simulink model "case7"  (R2024b)
settings: Solver=FixedStepAuto  StartTime=0  StopTime=1  FixedStep=1e-7  RelTol=1e-3
values from neighbouring files (symbols this model uses):
  SG_D_1_D = 0.01056    [IEEE9_case_parameters.m]    (also in case1_parameters.m; case2_parameters.m; case3_parameters.m; case4_parameters.m)
  SG_D_1_EnableSaturation = 0    [IEEE9_case_parameters.m]    (also in case1_parameters.m; case2_parameters.m; case3_parameters.m; case4_parameters.m)
  SG_D_1_f0 = 60    [IEEE9_case_parameters.m]    (also in case1_parameters.m; case2_parameters.m; case3_parameters.m; case4_parameters.m)
  SG_D_1_H = 7.5    [IEEE9_case_parameters.m]    (also in case1_parameters.m; case2_parameters.m; case3_parameters.m; case4_parameters.m)
  SG_D_1_K_A = 20    [IEEE9_case_parameters.m]    (also in case1_parameters.m; case2_parameters.m; case3_parameters.m; case4_parameters.m)
  SG_D_1_K_E = 1.000000e+1    (= 10)    [IEEE9_case_parameters.m]    (also in case1_parameters.m; case2_parameters.m; case3_parameters.m; case4_parameters.m)
  SG_D_1_K_F = 2.363    [IEEE9_case_parameters.m]    (also in case1_parameters.m; case2_parameters.m; case3_parameters.m; case4_parameters.m)
  SG_D_1_K_s = 0.5    [IEEE9_case_parameters.m]    (also in case1_parameters.m = 5; case2_parameters.m = 5; case3_parameters.m = 5; case4_parameters.m = 5)
  SG_D_1_R_a = 0.001088    [IEEE9_case_parameters.m]    (also in case1_parameters.m; case2_parameters.m; case3_parameters.m; case4_parameters.m)
  SG_D_1_S_A = 1    [IEEE9_case_parameters.m]    (also in case1_parameters.m; case2_parameters.m; case3_parameters.m; case4_parameters.m)
  SG_D_1_S_B = 0.103    [IEEE9_case_parameters.m]    (also in case1_parameters.m; case2_parameters.m; case3_parameters.m; case4_parameters.m)
  SG_D_1_S_N = 10.659857    [IEEE9_case_parameters.m]    (also in case1_parameters.m; case2_parameters.m; case3_parameters.m; case4_parameters.m)
  SG_D_1_SpeedPara = 200    [IEEE9_case_parameters.m]    (also in case1_parameters.m; case2_parameters.m; case3_parameters.m; case4_parameters.m)
  SG_D_1_T_0 = 0.720173    [IEEE9_case_parameters.m]    (also in case1_parameters.m = 0.755522; case2_parameters.m = 0.808931; case3_parameters.m = 0.869402; case4_parameters.m = 0.729316)
  SG_D_1_T_1 = 0.3    [IEEE9_case_parameters.m]    (also in case1_parameters.m; case2_parameters.m; case3_parameters.m; case4_parameters.m)
  SG_D_1_T_2 = 0.05    [IEEE9_case_parameters.m]    (also in case1_parameters.m; case2_parameters.m; case3_parameters.m; case4_parameters.m)
  SG_D_1_T_3 = 0.02    [IEEE9_case_parameters.m]    (also in case1_parameters.m; case2_parameters.m; case3_parameters.m; case4_parameters.m)
  SG_D_1_T_4 = 0.005    [IEEE9_case_parameters.m]    (also in case1_parameters.m; case2_parameters.m; case3_parameters.m; case4_parameters.m)
  SG_D_1_T_A = 0.02    [IEEE9_case_parameters.m]    (also in case1_parameters.m; case2_parameters.m; case3_parameters.m; case4_parameters.m)
  SG_D_1_T_dd = 8.000000e+0    (= 8)    [IEEE9_case_parameters.m]    (also in case1_parameters.m; case2_parameters.m; case3_parameters.m; case4_parameters.m)
  SG_D_1_T_ddd = 0.04    [IEEE9_case_parameters.m]    (also in case1_parameters.m; case2_parameters.m; case3_parameters.m; case4_parameters.m)
  SG_D_1_T_E = 0.314    [IEEE9_case_parameters.m]    (also in case1_parameters.m; case2_parameters.m; case3_parameters.m; case4_parameters.m)
  SG_D_1_T_F = 0.35    [IEEE9_case_parameters.m]    (also in case1_parameters.m; case2_parameters.m; case3_parameters.m; case4_parameters.m)
  SG_D_1_T_qd = 0.8    [IEEE9_case_parameters.m]    (also in case1_parameters.m; case2_parameters.m; case3_parameters.m; case4_parameters.m)
  SG_D_1_T_qdd = 0.02    [IEEE9_case_parameters.m]    (also in case1_parameters.m; case2_parameters.m; case3_parameters.m; case4_parameters.m)
  SG_D_1_T_speed = 0.1    [IEEE9_case_parameters.m]    (also in case1_parameters.m = 200; case2_parameters.m = 200; case3_parameters.m = 200; case4_parameters.m = 200)
  SG_D_1_T_w = 0.5    [IEEE9_case_parameters.m]    (also in case1_parameters.m; case2_parameters.m; case3_parameters.m; case4_parameters.m)
  SG_D_1_V_ref = 1.990276    [IEEE9_case_parameters.m]    (also in case1_parameters.m = 2.042296; case2_parameters.m = 2.051388; case3_parameters.m = 2.089584; case4_parameters.m = 2.01845)
  SG_D_1_w_ref = 376.991118    [IEEE9_case_parameters.m]    (also in case1_parameters.m; case2_parameters.m; case3_parameters.m; case4_parameters.m)
  SG_D_1_wb = 6.000000e+1    (= 60)    [IEEE9_case_parameters.m]    (also in case1_parameters.m; case2_parameters.m; case3_parameters.m; case4_parameters.m)
  SG_D_1_x_d = 1.9    [IEEE9_case_parameters.m]    (also in case1_parameters.m; case2_parameters.m; case3_parameters.m; case4_parameters.m)
  SG_D_1_x_dd = 0.302    [IEEE9_case_parameters.m]    (also in case1_parameters.m; case2_parameters.m; case3_parameters.m; case4_parameters.m)
  SG_D_1_x_ddd = 0.204    [IEEE9_case_parameters.m]    (also in case1_parameters.m; case2_parameters.m; case3_parameters.m; case4_parameters.m)
  SG_D_1_x_l = 0.05    [IEEE9_case_parameters.m]    (also in case1_parameters.m; case2_parameters.m; case3_parameters.m; case4_parameters.m)
  SG_D_1_x_q = 1.3    [IEEE9_case_parameters.m]    (also in case1_parameters.m; case2_parameters.m; case3_parameters.m; case4_parameters.m)
  SG_D_1_x_qd = 0.5    [IEEE9_case_parameters.m]    (also in case1_parameters.m; case2_parameters.m; case3_parameters.m; case4_parameters.m)
  SG_D_1_x_qdd = 0.3    [IEEE9_case_parameters.m]    (also in case1_parameters.m; case2_parameters.m; case3_parameters.m; case4_parameters.m)
  SG_D_2_D = 0.02    [IEEE9_case_parameters.m]    (also in case1_parameters.m; case2_parameters.m; case3_parameters.m; case4_parameters.m)
  SG_D_2_EnableSaturation = 0    [IEEE9_case_parameters.m]    (also in case1_parameters.m; case2_parameters.m; case3_parameters.m; case4_parameters.m)
  SG_D_2_f0 = 60    [IEEE9_case_parameters.m]    (also in case1_parameters.m; case2_parameters.m; case3_parameters.m; case4_parameters.m)
  SG_D_2_H = 8.000000e+0    (= 8)    [IEEE9_case_parameters.m]    (also in case1_parameters.m; case2_parameters.m; case3_parameters.m; case4_parameters.m)
  SG_D_2_K_A = 20    [IEEE9_case_parameters.m]    (also in case1_parameters.m; case2_parameters.m; case3_parameters.m; case4_parameters.m)
  SG_D_2_K_E = 1.000000e+1    (= 10)    [IEEE9_case_parameters.m]    (also in case1_parameters.m; case2_parameters.m; case3_parameters.m; case4_parameters.m)
  SG_D_2_K_F = 2.363    [IEEE9_case_parameters.m]    (also in case1_parameters.m; case2_parameters.m; case3_parameters.m; case4_parameters.m)
  SG_D_2_K_s = 0.5    [IEEE9_case_parameters.m]    (also in case1_parameters.m = 4; case2_parameters.m = 4; case3_parameters.m = 4; case4_parameters.m = 4)
  SG_D_2_R_a = 0.001088    [IEEE9_case_parameters.m]    (also in case1_parameters.m; case2_parameters.m; case3_parameters.m; case4_parameters.m)
  SG_D_2_S_A = 1    [IEEE9_case_parameters.m]    (also in case1_parameters.m; case2_parameters.m; case3_parameters.m; case4_parameters.m)
  SG_D_2_S_B = 0.103    [IEEE9_case_parameters.m]    (also in case1_parameters.m; case2_parameters.m; case3_parameters.m; case4_parameters.m)
  SG_D_2_S_N = 10.659857    [IEEE9_case_parameters.m]    (also in case1_parameters.m; case2_parameters.m; case3_parameters.m; case4_parameters.m)
  SG_D_2_SpeedPara = 200    [IEEE9_case_parameters.m]    (also in case1_parameters.m; case2_parameters.m; case3_parameters.m; case4_parameters.m)
  SG_D_2_T_0 = 1.632913    [IEEE9_case_parameters.m]    (also in case1_parameters.m = 1.632925; case2_parameters.m = 1.632915; case3_parameters.m = 1.632914; case4_parameters.m = 1.632927)
  SG_D_2_T_1 = 0.2    [IEEE9_case_parameters.m]    (also in case1_parameters.m; case2_parameters.m; case3_parameters.m; case4_parameters.m)
  SG_D_2_T_2 = 0.05    [IEEE9_case_parameters.m]    (also in case1_parameters.m; case2_parameters.m; case3_parameters.m; case4_parameters.m)
  SG_D_2_T_3 = 0.02    [IEEE9_case_parameters.m]    (also in case1_parameters.m; case2_parameters.m; case3_parameters.m; case4_parameters.m)
  SG_D_2_T_4 = 0.005    [IEEE9_case_parameters.m]    (also in case1_parameters.m; case2_parameters.m; case3_parameters.m; case4_parameters.m)
  SG_D_2_T_A = 0.02    [IEEE9_case_parameters.m]    (also in case1_parameters.m; case2_parameters.m; case3_parameters.m; case4_parameters.m)
  SG_D_2_T_dd = 7.9    [IEEE9_case_parameters.m]    (also in case1_parameters.m; case2_parameters.m; case3_parameters.m; case4_parameters.m)
  SG_D_2_T_ddd = 0.04    [IEEE9_case_parameters.m]    (also in case1_parameters.m; case2_parameters.m; case3_parameters.m; case4_parameters.m)
  SG_D_2_T_E = 0.314    [IEEE9_case_parameters.m]    (also in case1_parameters.m; case2_parameters.m; case3_parameters.m; case4_parameters.m)
  SG_D_2_T_F = 0.35    [IEEE9_case_parameters.m]    (also in case1_parameters.m; case2_parameters.m; case3_parameters.m; case4_parameters.m)
  SG_D_2_T_qd = 0.8    [IEEE9_case_parameters.m]    (also in case1_parameters.m; case2_parameters.m; case3_parameters.m; case4_parameters.m)
  SG_D_2_T_qdd = 0.015    [IEEE9_case_parameters.m]    (also in case1_parameters.m; case2_parameters.m; case3_parameters.m; case4_parameters.m)
  SG_D_2_T_speed = 0.1    [IEEE9_case_parameters.m]    (also in case1_parameters.m = 150; case2_parameters.m = 150; case3_parameters.m = 150; case4_parameters.m = 150)
  SG_D_2_T_w = 0.35    [IEEE9_case_parameters.m]    (also in case1_parameters.m; case2_parameters.m; case3_parameters.m; case4_parameters.m)
  SG_D_2_V_ref = 2.58547    [IEEE9_case_parameters.m]    (also in case1_parameters.m = 2.597896; case2_parameters.m = 2.587136; case3_parameters.m = 2.586042; case4_parameters.m = 2.599679)
  SG_D_2_w_ref = 376.991118    [IEEE9_case_parameters.m]    (also in case1_parameters.m; case2_parameters.m; case3_parameters.m; case4_parameters.m)
  SG_D_2_wb = 6.000000e+1    (= 60)    [IEEE9_case_parameters.m]    (also in case1_parameters.m; case2_parameters.m; case3_parameters.m; case4_parameters.m)
  SG_D_2_x_d = 1.8    [IEEE9_case_parameters.m]    (also in case1_parameters.m; case2_parameters.m; case3_parameters.m; case4_parameters.m)
  SG_D_2_x_dd = 0.302    [IEEE9_case_parameters.m]    (also in case1_parameters.m; case2_parameters.m; case3_parameters.m; case4_parameters.m)
  SG_D_2_x_ddd = 0.204    [IEEE9_case_parameters.m]    (also in case1_parameters.m; case2_parameters.m; case3_parameters.m; case4_parameters.m)
  SG_D_2_x_l = 0.05    [IEEE9_case_parameters.m]    (also in case1_parameters.m; case2_parameters.m; case3_parameters.m; case4_parameters.m)
  SG_D_2_x_q = 1.25    [IEEE9_case_parameters.m]    (also in case1_parameters.m; case2_parameters.m; case3_parameters.m; case4_parameters.m)
  SG_D_2_x_qd = 0.5    [IEEE9_case_parameters.m]    (also in case1_parameters.m; case2_parameters.m; case3_parameters.m; case4_parameters.m)
  SG_D_2_x_qdd = 0.3    [IEEE9_case_parameters.m]    (also in case1_parameters.m; case2_parameters.m; case3_parameters.m; case4_parameters.m)
  SG_D_3_D = 0.02    [IEEE9_case_parameters.m]    (also in case1_parameters.m; case2_parameters.m; case3_parameters.m; case4_parameters.m)
  SG_D_3_EnableSaturation = 0    [IEEE9_case_parameters.m]    (also in case1_parameters.m; case2_parameters.m; case3_parameters.m; case4_parameters.m)
  SG_D_3_f0 = 60    [IEEE9_case_parameters.m]    (also in case1_parameters.m; case2_parameters.m; case3_parameters.m; case4_parameters.m)
  SG_D_3_H = 7.7    [IEEE9_case_parameters.m]    (also in case1_parameters.m; case2_parameters.m; case3_parameters.m; case4_parameters.m)
  SG_D_3_K_A = 20    [IEEE9_case_parameters.m]    (also in case1_parameters.m; case2_parameters.m; case3_parameters.m; case4_parameters.m)
  SG_D_3_K_E = 1.000000e+1    (= 10)    [IEEE9_case_parameters.m]    (also in case1_parameters.m; case2_parameters.m; case3_parameters.m; case4_parameters.m)
  SG_D_3_K_F = 2.363    [IEEE9_case_parameters.m]    (also in case1_parameters.m; case2_parameters.m; case3_parameters.m; case4_parameters.m)
  SG_D_3_K_s = 0.2    [IEEE9_case_parameters.m]    (also in case1_parameters.m = 2; case2_parameters.m = 2; case3_parameters.m = 2; case4_parameters.m = 2)
  SG_D_3_R_a = 0.001088    [IEEE9_case_parameters.m]    (also in case1_parameters.m; case2_parameters.m; case3_parameters.m; case4_parameters.m)
  SG_D_3_S_A = 1    [IEEE9_case_parameters.m]    (also in case1_parameters.m; case2_parameters.m; case3_parameters.m; case4_parameters.m)
  SG_D_3_S_B = 0.103    [IEEE9_case_parameters.m]    (also in case1_parameters.m; case2_parameters.m; case3_parameters.m; case4_parameters.m)
  SG_D_3_S_N = 10.659857    [IEEE9_case_parameters.m]    (also in case1_parameters.m; case2_parameters.m; case3_parameters.m; case4_parameters.m)
  SG_D_3_SpeedPara = 200    [IEEE9_case_parameters.m]    (also in case1_parameters.m; case2_parameters.m; case3_parameters.m; case4_parameters.m)
  SG_D_3_T_0 = 0.850788    [IEEE9_case_parameters.m]    (also in case1_parameters.m = 0.850786; case2_parameters.m = 0.850787; case3_parameters.m; case4_parameters.m = 0.850786)
  SG_D_3_T_1 = 0.2    [IEEE9_case_parameters.m]    (also in case1_parameters.m; case2_parameters.m; case3_parameters.m; case4_parameters.m)
  SG_D_3_T_2 = 0.05    [IEEE9_case_parameters.m]    (also in case1_parameters.m; case2_parameters.m; case3_parameters.m; case4_parameters.m)
  SG_D_3_T_3 = 0.02    [IEEE9_case_parameters.m]    (also in case1_parameters.m; case2_parameters.m; case3_parameters.m; case4_parameters.m)
  SG_D_3_T_4 = 0.005    [IEEE9_case_parameters.m]    (also in case1_parameters.m; case2_parameters.m; case3_parameters.m; case4_parameters.m)
  SG_D_3_T_A = 0.02    [IEEE9_case_parameters.m]    (also in case1_parameters.m; case2_parameters.m; case3_parameters.m; case4_parameters.m)
  SG_D_3_T_dd = 8.1    [IEEE9_case_parameters.m]    (also in case1_parameters.m; case2_parameters.m; case3_parameters.m; case4_parameters.m)
  SG_D_3_T_ddd = 0.04    [IEEE9_case_parameters.m]    (also in case1_parameters.m; case2_parameters.m; case3_parameters.m; case4_parameters.m)
  SG_D_3_T_E = 0.314    [IEEE9_case_parameters.m]    (also in case1_parameters.m; case2_parameters.m; case3_parameters.m; case4_parameters.m)
  SG_D_3_T_F = 0.35    [IEEE9_case_parameters.m]    (also in case1_parameters.m; case2_parameters.m; case3_parameters.m; case4_parameters.m)
  SG_D_3_T_qd = 0.8    [IEEE9_case_parameters.m]    (also in case1_parameters.m; case2_parameters.m; case3_parameters.m; case4_parameters.m)
  SG_D_3_T_qdd = 0.015    [IEEE9_case_parameters.m]    (also in case1_parameters.m; case2_parameters.m; case3_parameters.m; case4_parameters.m)
  SG_D_3_T_speed = 0.1    [IEEE9_case_parameters.m]    (also in case1_parameters.m = 180; case2_parameters.m = 180; case3_parameters.m = 180; case4_parameters.m = 180)
  SG_D_3_T_w = 0.4    [IEEE9_case_parameters.m]    (also in case1_parameters.m; case2_parameters.m; case3_parameters.m; case4_parameters.m)
  SG_D_3_V_ref = 1.892727    [IEEE9_case_parameters.m]    (also in case1_parameters.m = 1.906439; case2_parameters.m = 1.895535; case3_parameters.m = 1.892105; case4_parameters.m = 1.906598)
  SG_D_3_w_ref = 376.991118    [IEEE9_case_parameters.m]    (also in case1_parameters.m; case2_parameters.m; case3_parameters.m; case4_parameters.m)
  SG_D_3_wb = 6.000000e+1    (= 60)    [IEEE9_case_parameters.m]    (also in case1_parameters.m; case2_parameters.m; case3_parameters.m; case4_parameters.m)
  SG_D_3_x_d = 1.85    [IEEE9_case_parameters.m]    (also in case1_parameters.m; case2_parameters.m; case3_parameters.m; case4_parameters.m)
  SG_D_3_x_dd = 0.302    [IEEE9_case_parameters.m]    (also in case1_parameters.m; case2_parameters.m; case3_parameters.m; case4_parameters.m)
  SG_D_3_x_ddd = 0.204    [IEEE9_case_parameters.m]    (also in case1_parameters.m; case2_parameters.m; case3_parameters.m; case4_parameters.m)
  SG_D_3_x_l = 0.05    [IEEE9_case_parameters.m]    (also in case1_parameters.m; case2_parameters.m; case3_parameters.m; case4_parameters.m)
  SG_D_3_x_q = 1.2    [IEEE9_case_parameters.m]    (also in case1_parameters.m; case2_parameters.m; case3_parameters.m; case4_parameters.m)
  SG_D_3_x_qd = 0.5    [IEEE9_case_parameters.m]    (also in case1_parameters.m; case2_parameters.m; case3_parameters.m; case4_parameters.m)
  SG_D_3_x_qdd = 0.3    [IEEE9_case_parameters.m]    (also in case1_parameters.m; case2_parameters.m; case3_parameters.m; case4_parameters.m)
(part 9 of 12)

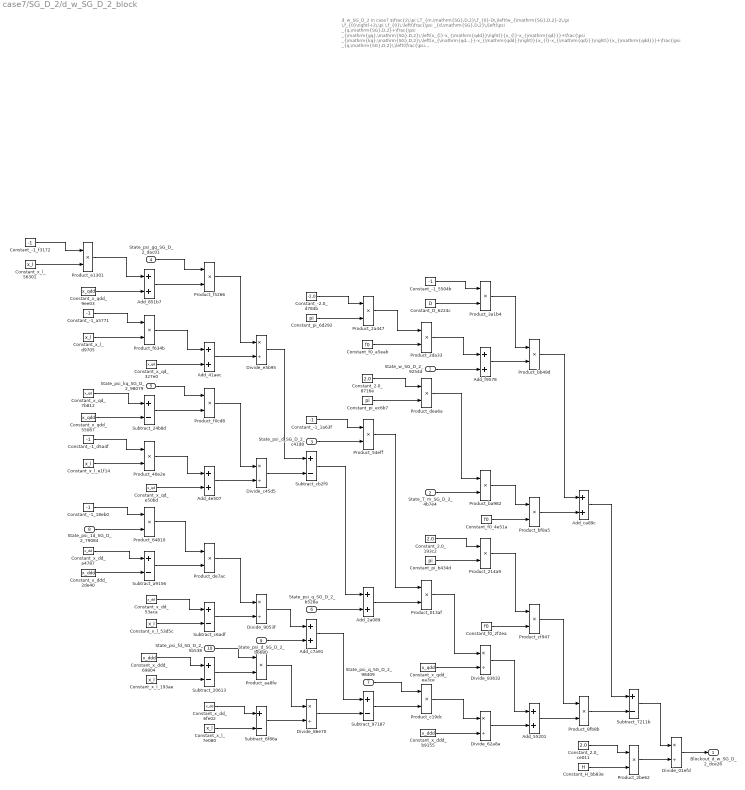
== system case7/SG_D_2/d_w_SG_D_2_block ==
  note: d_w_SG_D_2 in case7
      | $\frac{2\,\pi \,T_{m,\mathrm{SG},D,2}\,f_{0}-D\,\left(w_{\mathrm{SG},D,2}-2\,\pi \,f_{0}\right)+2\,\pi \,f_{0}\,\left(\frac{\psi _{d,\mathrm{SG},D,2}\,\left(\psi _{q,\mathrm{SG},D,2}+\frac{\psi _{\mathrm{gq},\mathrm{SG},D,2}\,\left(x_{l}-x_{\mathrm{qdd}}\right)}{x_{l}-x_{\mathrm{qd}}}+\frac{\psi _{\mathrm{kq},\mathrm{SG},D,2}\,\left(x_{\mathrm{qd}}-x_{\mathrm{qdd}}\right)}{x_{l}-x_{\mathrm{qd}}}\right)}{x_{\mathrm{qdd}}}+\frac{\psi _{q,\mathrm{SG},D,2}\,\left(\frac{\psi _{\mathrm{1d},\mathrm{SG},D,2}\,\left(x_{\mathrm{dd}}-x_{\mathrm{ddd}}\right)}{x_{\mathrm{dd}}-x_{l}}-\psi _{d,\mathrm{SG},D,2}+\frac{\psi _{\mathrm{fd},\mathrm{SG},D,2}\,\left(x_{\mathrm{ddd}}-x_{l}\right)}{x_{\mathrm{dd}}-x_{l}}\right)}{x_{\mathrm{ddd}}}\right)}{2\,H}$
      | Automatically generated on 2025-10-31 19:24:45 .
  State_w_SG_D_2_9254d : Inport
  State_T_m_SG_D_2_4b7e4 : Inport  Port=2
  State_psi_d_SG_D_2_c41d8 : Inport  Port=3
  State_psi_gq_SG_D_2_dac01 : Inport  Port=4
  State_psi_kq_SG_D_2_98079 : Inport  Port=5
  State_psi_q_SG_D_2_b528a : Inport  Port=6
  State_psi_q_SG_D_2_98409 : Inport  Port=7
  State_psi_1d_SG_D_2_79084 : Inport  Port=8
  State_psi_d_SG_D_2_b6680 : Inport  Port=9
  State_psi_fd_SG_D_2_5b538 : Inport  Port=10
  Add_2a089 : Sum
  Add_41aec : Sum
  Add_4e507 : Sum
  Add_55201 : Sum
  Add_851b7 : Sum
  Add_c7a91 : Sum
  Add_ca89c : Sum
  Add_f9578 : Sum
  Constant_-1_18eb0 : Constant  Value=-1
  Constant_-1_1a63f : Constant  Value=-1
  Constant_-1_5504b : Constant  Value=-1
  Constant_-1_a5771 : Constant  Value=-1
  Constant_-1_d5a4f : Constant  Value=-1
  Constant_-1_f3172 : Constant  Value=-1
  Constant_-2.0_d784b : Constant  Value=-2.0
  Constant_2.0_193c2 : Constant  Value=2.0
  Constant_2.0_8716e : Constant  Value=2.0
  Constant_2.0_ce011 : Constant  Value=2.0
  Constant_D_6224c : Constant  Value=D
  Constant_H_bb83e : Constant  Value=H
  Constant_f0_2f2ea : Constant  Value=f0
  Constant_f0_4e51a : Constant  Value=f0
  Constant_f0_a5eab : Constant  Value=f0
  Constant_pi_6d292 : Constant  Value=pi
  Constant_pi_b434d : Constant  Value=pi
  Constant_pi_ec6b7 : Constant  Value=pi
  Constant_x_dd_53aca : Constant  Value=x_dd
  Constant_x_dd_6fe02 : Constant  Value=x_dd
  Constant_x_dd_a4787 : Constant  Value=x_dd
  Constant_x_ddd_2de40 : Constant  Value=x_ddd
  Constant_x_ddd_69804 : Constant  Value=x_ddd
  Constant_x_ddd_b9155 : Constant  Value=x_ddd
  Constant_x_l_193ae : Constant  Value=x_l
  Constant_x_l_53d5c : Constant  Value=x_l
  Constant_x_l_56301 : Constant  Value=x_l
  Constant_x_l_7e080 : Constant  Value=x_l
  Constant_x_l_d9705 : Constant  Value=x_l
  Constant_x_l_e1f14 : Constant  Value=x_l
  Constant_x_qd_327e0 : Constant  Value=x_qd
  Constant_x_qd_7b812 : Constant  Value=x_qd
  Constant_x_qd_e50bd : Constant  Value=x_qd
  Constant_x_qdd_55067 : Constant  Value=x_qdd
  Constant_x_qdd_9ee03 : Constant  Value=x_qdd
  Constant_x_qdd_ea3ce : Constant  Value=x_qdd
  Divide_01efd : Product  Inputs=*/
  Divide_62a8a : Product  Inputs=*/
  Divide_83632 : Product  Inputs=*/
  Divide_86e70 : Product  Inputs=*/
  Divide_9053f : Product  Inputs=*/
  Divide_c45d5 : Product  Inputs=*/
  Divide_e5b95 : Product  Inputs=*/
  Product_013af : Product
  Product_214a9 : Product
  Product_2a447 : Product
  Product_2be62 : Product
  Product_2da33 : Product
  Product_3a1b4 : Product
  Product_40e2e : Product
  Product_54eff : Product
  Product_64810 : Product
  Product_8fb8b : Product
  Product_aa8fe : Product
  Product_ba982 : Product
  Product_bb49d : Product
  Product_bf8a5 : Product
  Product_c19dc : Product
  Product_cf947 : Product
  Product_de7ac : Product
  Product_dea6a : Product
  Product_e1301 : Product
  Product_f0cd8 : Product
  Product_f5266 : Product
  Product_f634b : Product
  Subtract_20613 : Sum  Inputs=+-
  Subtract_24b8d : Sum  Inputs=+-
  Subtract_6f86a : Sum  Inputs=+-
  Subtract_7211b : Sum  Inputs=+-
  Subtract_97187 : Sum  Inputs=+-
  Subtract_a9156 : Sum  Inputs=+-
  Subtract_c6adf : Sum  Inputs=+-
  Subtract_cb2f9 : Sum  Inputs=+-
  Blockout_d_w_SG_D_2_dce26 : Outport
  wires:
  Constant_x_qd_7b812/1 -> Subtract_24b8d/1
  Constant_-1_d5a4f/1 -> Product_40e2e/1
  Constant_-1_f3172/1 -> Product_e1301/1
  Constant_x_qdd_55067/1 -> Subtract_24b8d/2
  Subtract_6f86a/1 -> Divide_86e70/2
  Constant_x_l_e1f14/1 -> Product_40e2e/2
  Constant_x_l_56301/1 -> Product_e1301/2
  Product_40e2e/1 -> Add_4e507/1
  Product_e1301/1 -> Add_851b7/1
  Constant_x_l_53d5c/1 -> Subtract_c6adf/2
  Constant_x_l_d9705/1 -> Product_f634b/2
  Constant_x_ddd_b9155/1 -> Divide_62a8a/2
  Subtract_20613/1 -> Product_aa8fe/2
  Constant_x_qd_e50bd/1 -> Add_4e507/2
  Constant_x_qdd_9ee03/1 -> Add_851b7/2
  Constant_-1_a5771/1 -> Product_f634b/1
  State_psi_d_SG_D_2_c41d8/1 -> Product_54eff/2
  Constant_-1_18eb0/1 -> Product_64810/1
  State_w_SG_D_2_9254d/1 -> Add_f9578/2
  Product_f634b/1 -> Add_41aec/1
  State_psi_1d_SG_D_2_79084/1 -> Product_64810/2
  Constant_x_dd_a4787/1 -> Subtract_a9156/1
  Divide_e5b95/1 -> Subtract_cb2f9/1
  Subtract_24b8d/1 -> Product_f0cd8/2
  Constant_x_ddd_2de40/1 -> Subtract_a9156/2
  State_psi_gq_SG_D_2_dac01/1 -> Product_f5266/1
  Add_4e507/1 -> Divide_c45d5/2
  State_psi_d_SG_D_2_b6680/1 -> Add_c7a91/2
  Add_851b7/1 -> Product_f5266/2
  Constant_x_qd_327e0/1 -> Add_41aec/2
  State_psi_kq_SG_D_2_98079/1 -> Product_f0cd8/1
  Product_64810/1 -> Product_de7ac/1
  Subtract_a9156/1 -> Product_de7ac/2
  Constant_pi_ec6b7/1 -> Product_dea6a/2
  Constant_x_dd_53aca/1 -> Subtract_c6adf/1
  Constant_x_ddd_69804/1 -> Subtract_20613/1
  Constant_x_l_193ae/1 -> Subtract_20613/2
  Product_f5266/1 -> Divide_e5b95/1
  Add_41aec/1 -> Divide_e5b95/2
  Add_2a089/1 -> Product_013af/2
  Product_f0cd8/1 -> Divide_c45d5/1
  Constant_pi_6d292/1 -> Product_2a447/2
  Product_de7ac/1 -> Divide_9053f/1
  Subtract_c6adf/1 -> Divide_9053f/2
  State_psi_fd_SG_D_2_5b538/1 -> Product_aa8fe/1
  Divide_9053f/1 -> Add_c7a91/1
  Constant_x_dd_6fe02/1 -> Subtract_6f86a/1
  Constant_x_l_7e080/1 -> Subtract_6f86a/2
  Divide_c45d5/1 -> Subtract_cb2f9/2
  Product_aa8fe/1 -> Divide_86e70/1
  Constant_-1_1a63f/1 -> Product_54eff/1
  Constant_-2.0_d784b/1 -> Product_2a447/1
  Subtract_cb2f9/1 -> Add_2a089/1
  Subtract_97187/1 -> Product_c19dc/2
  State_psi_q_SG_D_2_b528a/1 -> Add_2a089/2
  Constant_D_6224c/1 -> Product_3a1b4/2
  Add_c7a91/1 -> Subtract_97187/1
  Divide_86e70/1 -> Subtract_97187/2
  Product_2a447/1 -> Product_2da33/1
  Constant_f0_a5eab/1 -> Product_2da33/2
  Constant_2.0_8716e/1 -> Product_dea6a/1
  Product_54eff/1 -> Product_013af/1
  State_psi_q_SG_D_2_98409/1 -> Product_c19dc/1
  Constant_-1_5504b/1 -> Product_3a1b4/1
  Product_2da33/1 -> Add_f9578/1
  Product_dea6a/1 -> Product_ba982/1
  State_T_m_SG_D_2_4b7e4/1 -> Product_ba982/2
  Constant_2.0_193c2/1 -> Product_214a9/1
  Constant_pi_b434d/1 -> Product_214a9/2
  Product_013af/1 -> Divide_83632/1
  Constant_x_qdd_ea3ce/1 -> Divide_83632/2
  Product_c19dc/1 -> Divide_62a8a/1
  Product_3a1b4/1 -> Product_bb49d/1
  Add_f9578/1 -> Product_bb49d/2
  Product_ba982/1 -> Product_bf8a5/1
  Constant_f0_4e51a/1 -> Product_bf8a5/2
  Product_214a9/1 -> Product_cf947/1
  Constant_f0_2f2ea/1 -> Product_cf947/2
  Divide_83632/1 -> Add_55201/1
  Divide_62a8a/1 -> Add_55201/2
  Product_bb49d/1 -> Add_ca89c/1
  Product_bf8a5/1 -> Add_ca89c/2
  Product_cf947/1 -> Product_8fb8b/1
  Add_55201/1 -> Product_8fb8b/2
  Add_ca89c/1 -> Subtract_7211b/1
  Product_8fb8b/1 -> Subtract_7211b/2
  Constant_2.0_ce011/1 -> Product_2be62/1
  Constant_H_bb83e/1 -> Product_2be62/2
  Subtract_7211b/1 -> Divide_01efd/1
  Product_2be62/1 -> Divide_01efd/2
  Divide_01efd/1 -> Blockout_d_w_SG_D_2_dce26/1

== system case7/SG_D_2/i_d_SG_D_2_block ==
  note: i_d_SG_D_2 in case7
      | $\frac{\sin\left(\theta _{\mathrm{SG},D,2}\right)\,\left(\frac{\psi _{\mathrm{1d},\mathrm{SG},D,2}\,\left(x_{\mathrm{dd}}-x_{\mathrm{ddd}}\right)}{x_{\mathrm{dd}}-x_{l}}-\psi _{d,\mathrm{SG},D,2}+\frac{\psi _{\mathrm{fd},\mathrm{SG},D,2}\,\left(x_{\mathrm{ddd}}-x_{l}\right)}{x_{\mathrm{dd}}-x_{l}}\right)}{x_{\mathrm{ddd}}}-\frac{\cos\left(\theta _{\mathrm{SG},D,2}\right)\,\left(\psi _{q,\mathrm{SG},D,2}+\frac{\psi _{\mathrm{gq},\mathrm{SG},D,2}\,\left(x_{l}-x_{\mathrm{qdd}}\right)}{x_{l}-x_{\mathrm{qd}}}+\frac{\psi _{\mathrm{kq},\mathrm{SG},D,2}\,\left(x_{\mathrm{qd}}-x_{\mathrm{qdd}}\right)}{x_{l}-x_{\mathrm{qd}}}\right)}{x_{\mathrm{qdd}}}$
      | Automatically generated on 2025-10-31 19:25:10 .
  State_psi_gq_SG_D_2_2ca68 : Inport
  State_psi_kq_SG_D_2_f7ad5 : Inport  Port=2
  State_psi_q_SG_D_2_5a7c7 : Inport  Port=3
  State_theta_SG_D_2_df193 : Inport  Port=4
  State_psi_1d_SG_D_2_3541a : Inport  Port=5
  State_psi_d_SG_D_2_d4d6e : Inport  Port=6
  State_psi_fd_SG_D_2_e8aea : Inport  Port=7
  State_theta_SG_D_2_1457d : Inport  Port=8
  Add_02f62 : Sum
  Add_0cd5c : Sum
  Add_a7fd3 : Sum
  Add_dcc12 : Sum
  Add_f66c1 : Sum
  Constant_-1_29c56 : Constant  Value=-1
  Constant_-1_5d0ed : Constant  Value=-1
  Constant_-1_62571 : Constant  Value=-1
  Constant_-1_8b6c8 : Constant  Value=-1
  Constant_-1_d679d : Constant  Value=-1
  Constant_x_dd_28971 : Constant  Value=x_dd
  Constant_x_dd_ae3c7 : Constant  Value=x_dd
  Constant_x_dd_ead17 : Constant  Value=x_dd
  Constant_x_ddd_add92 : Constant  Value=x_ddd
  Constant_x_ddd_ae131 : Constant  Value=x_ddd
  Constant_x_ddd_cd715 : Constant  Value=x_ddd
  Constant_x_l_43de9 : Constant  Value=x_l
  Constant_x_l_4e15d : Constant  Value=x_l
  Constant_x_l_6490b : Constant  Value=x_l
  Constant_x_l_a8adc : Constant  Value=x_l
  Constant_x_l_b12d3 : Constant  Value=x_l
  Constant_x_l_ef573 : Constant  Value=x_l
  Constant_x_qd_2ed36 : Constant  Value=x_qd
  Constant_x_qd_372c2 : Constant  Value=x_qd
  Constant_x_qd_7e301 : Constant  Value=x_qd
  Constant_x_qdd_68186 : Constant  Value=x_qdd
  Constant_x_qdd_7ddfe : Constant  Value=x_qdd
  Constant_x_qdd_81e8f : Constant  Value=x_qdd
  Divide_23844 : Product  Inputs=*/
  Divide_38aa0 : Product  Inputs=*/
  Divide_419be : Product  Inputs=*/
  Divide_52d14 : Product  Inputs=*/
  Divide_578a3 : Product  Inputs=*/
  Divide_c5ebf : Product  Inputs=*/
  MathFunc_cos_b87ab : Trigonometry  Operator=cos
  MathFunc_sin_26994 : Trigonometry
  Product_06a70 : Product
  Product_1f7d0 : Product
  Product_21f17 : Product
  Product_32eeb : Product
  Product_43aee : Product
  Product_5dae6 : Product
  Product_76d2a : Product
  Product_9c28c : Product
  Product_a6e65 : Product
  Product_d9ed7 : Product
  Product_e7dc2 : Product
  Subtract_5c624 : Sum  Inputs=+-
  Subtract_755a9 : Sum  Inputs=+-
  Subtract_76564 : Sum  Inputs=+-
  Subtract_aaaa7 : Sum  Inputs=+-
  Subtract_b0076 : Sum  Inputs=+-
  Subtract_d04c5 : Sum  Inputs=+-
  Subtract_f9caf : Sum  Inputs=+-
  Subtract_fa517 : Sum  Inputs=+-
  Blockout_i_d_SG_D_2_adf62 : Outport
  wires:
  Constant_x_ddd_cd715/1 -> Subtract_5c624/1
  Constant_x_qd_2ed36/1 -> Subtract_76564/1
  Constant_-1_8b6c8/1 -> Product_06a70/1
  Constant_-1_62571/1 -> Product_a6e65/1
  Subtract_d04c5/1 -> Blockout_i_d_SG_D_2_adf62/1
  Constant_x_qdd_68186/1 -> Subtract_76564/2
  Constant_x_l_6490b/1 -> Product_06a70/2
  Constant_x_l_b12d3/1 -> Product_a6e65/2
  Product_06a70/1 -> Add_a7fd3/1
  Product_a6e65/1 -> Add_02f62/1
  Constant_x_l_43de9/1 -> Product_5dae6/2
  Constant_x_qd_372c2/1 -> Add_a7fd3/2
  Constant_x_qdd_81e8f/1 -> Add_02f62/2
  Constant_x_qdd_7ddfe/1 -> Divide_38aa0/2
  MathFunc_cos_b87ab/1 -> Product_9c28c/2
  Constant_-1_d679d/1 -> Product_5dae6/1
  State_psi_gq_SG_D_2_2ca68/1 -> Product_43aee/1
  Subtract_5c624/1 -> Product_e7dc2/2
  Product_1f7d0/1 -> Product_76d2a/1
  Add_a7fd3/1 -> Divide_23844/2
  Add_02f62/1 -> Product_43aee/2
  Product_e7dc2/1 -> Divide_c5ebf/1
  Product_5dae6/1 -> Add_dcc12/1
  Constant_x_qd_7e301/1 -> Add_dcc12/2
  State_theta_SG_D_2_1457d/1 -> MathFunc_sin_26994/1
  State_psi_kq_SG_D_2_f7ad5/1 -> Product_21f17/1
  Add_f66c1/1 -> Subtract_fa517/1
  Subtract_76564/1 -> Product_21f17/2
  Product_43aee/1 -> Divide_419be/1
  Constant_-1_29c56/1 -> Product_1f7d0/1
  State_psi_1d_SG_D_2_3541a/1 -> Product_1f7d0/2
  State_psi_fd_SG_D_2_e8aea/1 -> Product_e7dc2/1
  Constant_x_dd_28971/1 -> Subtract_b0076/1
  Product_76d2a/1 -> Divide_578a3/1
  Constant_x_ddd_add92/1 -> Subtract_b0076/2
  Divide_c5ebf/1 -> Subtract_fa517/2
  Add_dcc12/1 -> Divide_419be/2
  Product_32eeb/1 -> Divide_52d14/1
  Product_21f17/1 -> Divide_23844/1
  Constant_-1_5d0ed/1 -> Product_d9ed7/1
  Subtract_f9caf/1 -> Divide_c5ebf/2
  Subtract_b0076/1 -> Product_76d2a/2
  Constant_x_dd_ead17/1 -> Subtract_aaaa7/1
  Subtract_fa517/1 -> Product_32eeb/1
  Constant_x_l_ef573/1 -> Subtract_aaaa7/2
  Constant_x_l_4e15d/1 -> Subtract_5c624/2
  Divide_419be/1 -> Subtract_755a9/1
  Divide_52d14/1 -> Subtract_d04c5/2
  Divide_23844/1 -> Subtract_755a9/2
  Subtract_aaaa7/1 -> Divide_578a3/2
  Constant_x_dd_ae3c7/1 -> Subtract_f9caf/1
  Divide_38aa0/1 -> Subtract_d04c5/1
  Constant_x_l_a8adc/1 -> Subtract_f9caf/2
  Subtract_755a9/1 -> Add_0cd5c/1
  State_psi_q_SG_D_2_5a7c7/1 -> Add_0cd5c/2
  Constant_x_ddd_ae131/1 -> Divide_52d14/2
  MathFunc_sin_26994/1 -> Product_32eeb/2
  Divide_578a3/1 -> Add_f66c1/1
  State_psi_d_SG_D_2_d4d6e/1 -> Add_f66c1/2
  Add_0cd5c/1 -> Product_d9ed7/2
  State_theta_SG_D_2_df193/1 -> MathFunc_cos_b87ab/1
  Product_d9ed7/1 -> Product_9c28c/1
  Product_9c28c/1 -> Divide_38aa0/1

== system case7/SG_D_2/i_q_SG_D_2_block ==
  note: i_q_SG_D_2 in case7
      | $-\frac{\sin\left(\theta _{\mathrm{SG},D,2}\right)\,\left(\psi _{q,\mathrm{SG},D,2}+\frac{\psi _{\mathrm{gq},\mathrm{SG},D,2}\,\left(x_{l}-x_{\mathrm{qdd}}\right)}{x_{l}-x_{\mathrm{qd}}}+\frac{\psi _{\mathrm{kq},\mathrm{SG},D,2}\,\left(x_{\mathrm{qd}}-x_{\mathrm{qdd}}\right)}{x_{l}-x_{\mathrm{qd}}}\right)}{x_{\mathrm{qdd}}}-\frac{\cos\left(\theta _{\mathrm{SG},D,2}\right)\,\left(\frac{\psi _{\mathrm{1d},\mathrm{SG},D,2}\,\left(x_{\mathrm{dd}}-x_{\mathrm{ddd}}\right)}{x_{\mathrm{dd}}-x_{l}}-\psi _{d,\mathrm{SG},D,2}+\frac{\psi _{\mathrm{fd},\mathrm{SG},D,2}\,\left(x_{\mathrm{ddd}}-x_{l}\right)}{x_{\mathrm{dd}}-x_{l}}\right)}{x_{\mathrm{ddd}}}$
      | Automatically generated on 2025-10-31 19:25:15 .
  State_psi_gq_SG_D_2_9874f : Inport
  State_psi_kq_SG_D_2_111a7 : Inport  Port=2
  State_psi_q_SG_D_2_3ac1e : Inport  Port=3
  State_theta_SG_D_2_a60df : Inport  Port=4
  State_psi_1d_SG_D_2_f6d17 : Inport  Port=5
  State_psi_d_SG_D_2_87493 : Inport  Port=6
  State_psi_fd_SG_D_2_e2311 : Inport  Port=7
  State_theta_SG_D_2_15c5e : Inport  Port=8
  Add_47226 : Sum
  Add_5ccf0 : Sum
  Add_a14e2 : Sum
  Add_a2117 : Sum
  Add_b99c9 : Sum
  Add_fc011 : Sum
  Constant_-1_7f3d5 : Constant  Value=-1
  Constant_-1_9c186 : Constant  Value=-1
  Constant_-1_c7991 : Constant  Value=-1
  Constant_-1_dccd0 : Constant  Value=-1
  Constant_-1_e85db : Constant  Value=-1
  Constant_x_dd_1673e : Constant  Value=x_dd
  Constant_x_dd_32dbf : Constant  Value=x_dd
  Constant_x_dd_f85f6 : Constant  Value=x_dd
  Constant_x_ddd_38ac4 : Constant  Value=x_ddd
  Constant_x_ddd_9e79b : Constant  Value=x_ddd
  Constant_x_ddd_b931f : Constant  Value=x_ddd
  Constant_x_l_06c4d : Constant  Value=x_l
  Constant_x_l_152f5 : Constant  Value=x_l
  Constant_x_l_3ea75 : Constant  Value=x_l
  Constant_x_l_6f93f : Constant  Value=x_l
  Constant_x_l_c61d2 : Constant  Value=x_l
  Constant_x_l_d95ac : Constant  Value=x_l
  Constant_x_qd_2f00b : Constant  Value=x_qd
  Constant_x_qd_36ab8 : Constant  Value=x_qd
  Constant_x_qd_e8c91 : Constant  Value=x_qd
  Constant_x_qdd_2eeb8 : Constant  Value=x_qdd
  Constant_x_qdd_9ffa4 : Constant  Value=x_qdd
  Constant_x_qdd_fe3a8 : Constant  Value=x_qdd
  Divide_0e3e2 : Product  Inputs=*/
  Divide_3840a : Product  Inputs=*/
  Divide_5cecb : Product  Inputs=*/
  Divide_7c5c9 : Product  Inputs=*/
  Divide_a04bd : Product  Inputs=*/
  Divide_cc190 : Product  Inputs=*/
  MathFunc_cos_6cc96 : Trigonometry  Operator=cos
  MathFunc_sin_f19d1 : Trigonometry
  Product_0501a : Product
  Product_174c4 : Product
  Product_1cb07 : Product
  Product_30e2b : Product
  Product_528d3 : Product
  Product_5584f : Product
  Product_6f1f7 : Product
  Product_841b9 : Product
  Product_af52f : Product
  Product_bef50 : Product
  Product_e3c35 : Product
  Subtract_72183 : Sum  Inputs=+-
  Subtract_7a1d9 : Sum  Inputs=+-
  Subtract_8e66a : Sum  Inputs=+-
  Subtract_976aa : Sum  Inputs=+-
  Subtract_cfac8 : Sum  Inputs=+-
  Subtract_eb1ff : Sum  Inputs=+-
  Subtract_fdf02 : Sum  Inputs=+-
  Blockout_i_q_SG_D_2_2255f : Outport
  wires:
  MathFunc_sin_f19d1/1 -> Product_841b9/2
  Product_30e2b/1 -> Product_841b9/1
  Constant_-1_9c186/1 -> Product_6f1f7/1
  Constant_-1_e85db/1 -> Product_1cb07/1
  Constant_x_l_3ea75/1 -> Product_6f1f7/2
  Product_6f1f7/1 -> Add_fc011/1
  Subtract_7a1d9/1 -> Product_5584f/2
  Constant_x_qdd_9ffa4/1 -> Subtract_cfac8/2
  Constant_x_qdd_fe3a8/1 -> Add_fc011/2
  Add_a2117/1 -> Product_30e2b/2
  Constant_x_l_152f5/1 -> Product_1cb07/2
  Constant_x_qd_e8c91/1 -> Subtract_cfac8/1
  Constant_-1_7f3d5/1 -> Product_528d3/1
  Constant_x_l_d95ac/1 -> Product_528d3/2
  State_psi_1d_SG_D_2_f6d17/1 -> Product_0501a/2
  State_psi_gq_SG_D_2_9874f/1 -> Product_e3c35/1
  Add_fc011/1 -> Product_e3c35/2
  Product_1cb07/1 -> Add_b99c9/1
  Divide_0e3e2/1 -> Add_a14e2/1
  Constant_x_qd_36ab8/1 -> Add_b99c9/2
  State_psi_kq_SG_D_2_111a7/1 -> Product_af52f/1
  Add_47226/1 -> Subtract_72183/1
  Constant_x_ddd_b931f/1 -> Subtract_7a1d9/2
  Subtract_cfac8/1 -> Product_af52f/2
  Product_528d3/1 -> Add_5ccf0/1
  Constant_x_qd_2f00b/1 -> Add_5ccf0/2
  Constant_-1_dccd0/1 -> Product_0501a/1
  Constant_x_l_06c4d/1 -> Subtract_fdf02/2
  Constant_x_dd_32dbf/1 -> Subtract_7a1d9/1
  Product_e3c35/1 -> Divide_5cecb/1
  Divide_a04bd/1 -> Subtract_72183/2
  Add_b99c9/1 -> Divide_5cecb/2
  Product_bef50/1 -> Divide_7c5c9/1
  Product_af52f/1 -> Divide_3840a/1
  Constant_-1_c7991/1 -> Product_30e2b/1
  Product_0501a/1 -> Product_5584f/1
  Add_5ccf0/1 -> Divide_3840a/2
  Constant_x_dd_f85f6/1 -> Subtract_eb1ff/1
  Subtract_72183/1 -> Product_bef50/1
  Subtract_8e66a/1 -> Product_174c4/2
  Constant_x_l_c61d2/1 -> Subtract_eb1ff/2
  Constant_x_ddd_9e79b/1 -> Subtract_8e66a/1
  Constant_x_l_6f93f/1 -> Subtract_8e66a/2
  Divide_5cecb/1 -> Subtract_976aa/1
  Divide_7c5c9/1 -> Add_a14e2/2
  Product_174c4/1 -> Divide_a04bd/1
  Divide_3840a/1 -> Subtract_976aa/2
  Subtract_fdf02/1 -> Divide_a04bd/2
  Product_5584f/1 -> Divide_cc190/1
  Subtract_eb1ff/1 -> Divide_cc190/2
  Constant_x_qdd_2eeb8/1 -> Divide_0e3e2/2
  State_psi_fd_SG_D_2_e2311/1 -> Product_174c4/1
  Constant_x_dd_1673e/1 -> Subtract_fdf02/1
  Subtract_976aa/1 -> Add_a2117/1
  State_psi_q_SG_D_2_3ac1e/1 -> Add_a2117/2
  Constant_x_ddd_38ac4/1 -> Divide_7c5c9/2
  Divide_cc190/1 -> Add_47226/1
  State_psi_d_SG_D_2_87493/1 -> Add_47226/2
  State_theta_SG_D_2_a60df/1 -> MathFunc_sin_f19d1/1
  State_theta_SG_D_2_15c5e/1 -> MathFunc_cos_6cc96/1
  MathFunc_cos_6cc96/1 -> Product_bef50/2
  Product_841b9/1 -> Divide_0e3e2/1
  Add_a14e2/1 -> Blockout_i_q_SG_D_2_2255f/1

== system case7/SG_D_2/theta_SG_D_2_out_block ==
  note: theta_SG_D_2_out in case7
      | $\theta _{\mathrm{SG},D,2}$
      | Automatically generated on 2025-10-31 19:25:21 .
  State_theta_SG_D_2_7f9e2 : Inport
  Blockout_theta_SG_D_2_out_31e40 : Outport
  wires:
  State_theta_SG_D_2_7f9e2/1 -> Blockout_theta_SG_D_2_out_31e40/1

== system case7/SG_D_2/w_SG_D_2_out_block ==
  note: w_SG_D_2_out in case7
      | $w_{\mathrm{SG},D,2}$
      | Automatically generated on 2025-10-31 19:25:21 .
  State_w_SG_D_2_7ae1a : Inport
  Blockout_w_SG_D_2_out_61ea1 : Outport
  wires:
  State_w_SG_D_2_7ae1a/1 -> Blockout_w_SG_D_2_out_61ea1/1

== system case7/SG_D_3/T_e_SG_D_3_block ==
  note: T_e_SG_D_3 in case7
      | $-\frac{\psi _{d,\mathrm{SG},D,3}\,\left(\psi _{q,\mathrm{SG},D,3}+\frac{\psi _{\mathrm{gq},\mathrm{SG},D,3}\,\left(x_{l}-x_{\mathrm{qdd}}\right)}{x_{l}-x_{\mathrm{qd}}}+\frac{\psi _{\mathrm{kq},\mathrm{SG},D,3}\,\left(x_{\mathrm{qd}}-x_{\mathrm{qdd}}\right)}{x_{l}-x_{\mathrm{qd}}}\right)}{x_{\mathrm{qdd}}}-\frac{\psi _{q,\mathrm{SG},D,3}\,\left(\frac{\psi _{\mathrm{1d},\mathrm{SG},D,3}\,\left(x_{\mathrm{dd}}-x_{\mathrm{ddd}}\right)}{x_{\mathrm{dd}}-x_{l}}-\psi _{d,\mathrm{SG},D,3}+\frac{\psi _{\mathrm{fd},\mathrm{SG},D,3}\,\left(x_{\mathrm{ddd}}-x_{l}\right)}{x_{\mathrm{dd}}-x_{l}}\right)}{x_{\mathrm{ddd}}}$
      | Automatically generated on 2025-10-31 19:26:39 .
  State_psi_d_SG_D_3_21043 : Inport
  State_psi_gq_SG_D_3_33d2c : Inport  Port=2
  State_psi_kq_SG_D_3_78f61 : Inport  Port=3
  State_psi_q_SG_D_3_08b99 : Inport  Port=4
  State_psi_q_SG_D_3_6cef3 : Inport  Port=5
  State_psi_1d_SG_D_3_4e6ed : Inport  Port=6
  State_psi_d_SG_D_3_2ba64 : Inport  Port=7
  State_psi_fd_SG_D_3_03760 : Inport  Port=8
  Add_4be3a : Sum
  Add_52871 : Sum
  Add_5537a : Sum
  Add_9b82a : Sum
  Add_ba54b : Sum
  Add_d82aa : Sum
  Constant_-1_1a5f0 : Constant  Value=-1
  Constant_-1_2ecb7 : Constant  Value=-1
  Constant_-1_3da43 : Constant  Value=-1
  Constant_-1_4525a : Constant  Value=-1
  Constant_-1_81735 : Constant  Value=-1
  Constant_x_dd_2b2ae : Constant  Value=x_dd
  Constant_x_dd_9bd23 : Constant  Value=x_dd
  Constant_x_dd_ff414 : Constant  Value=x_dd
  Constant_x_ddd_00f81 : Constant  Value=x_ddd
  Constant_x_ddd_a9188 : Constant  Value=x_ddd
  Constant_x_ddd_f68ef : Constant  Value=x_ddd
  Constant_x_l_114b1 : Constant  Value=x_l
  Constant_x_l_2b5e6 : Constant  Value=x_l
  Constant_x_l_58231 : Constant  Value=x_l
  Constant_x_l_583f1 : Constant  Value=x_l
  Constant_x_l_b5fbc : Constant  Value=x_l
  Constant_x_l_f3b31 : Constant  Value=x_l
  Constant_x_qd_55fd7 : Constant  Value=x_qd
  Constant_x_qd_c058a : Constant  Value=x_qd
  Constant_x_qd_eba46 : Constant  Value=x_qd
  Constant_x_qdd_73938 : Constant  Value=x_qdd
  Constant_x_qdd_d5a40 : Constant  Value=x_qdd
  Constant_x_qdd_d6058 : Constant  Value=x_qdd
  Divide_0d433 : Product  Inputs=*/
  Divide_2e403 : Product  Inputs=*/
  Divide_4b437 : Product  Inputs=*/
  Divide_51fce : Product  Inputs=*/
  Divide_d1542 : Product  Inputs=*/
  Divide_f1a46 : Product  Inputs=*/
  Product_07c94 : Product
  Product_16dfe : Product
  Product_3102b : Product
  Product_3863b : Product
  Product_40773 : Product
  Product_4afca : Product
  Product_67516 : Product
  Product_7b82c : Product
  Product_8cdad : Product
  Product_ae01e : Product
  Product_f93d2 : Product
  Subtract_0262a : Sum  Inputs=+-
  Subtract_02e5a : Sum  Inputs=+-
  Subtract_1ae10 : Sum  Inputs=+-
  Subtract_277e5 : Sum  Inputs=+-
  Subtract_ad55d : Sum  Inputs=+-
  Subtract_cb1bc : Sum  Inputs=+-
  Subtract_cc85e : Sum  Inputs=+-
  Blockout_T_e_SG_D_3_4c18a : Outport
  wires:
  State_psi_q_SG_D_3_08b99/1 -> Add_d82aa/2
  Constant_-1_4525a/1 -> Product_ae01e/1
  Subtract_1ae10/1 -> Product_4afca/2
  State_psi_1d_SG_D_3_4e6ed/1 -> Product_3863b/2
  Constant_-1_2ecb7/1 -> Product_67516/1
  Constant_x_l_583f1/1 -> Product_67516/2
  Add_ba54b/1 -> Subtract_1ae10/1
  State_psi_d_SG_D_3_2ba64/1 -> Add_ba54b/2
  Product_67516/1 -> Add_4be3a/1
  Constant_x_qdd_d5a40/1 -> Subtract_02e5a/2
  Add_d82aa/1 -> Product_7b82c/2
  Constant_x_qdd_d6058/1 -> Add_4be3a/2
  State_psi_q_SG_D_3_6cef3/1 -> Product_4afca/1
  Constant_x_l_114b1/1 -> Product_ae01e/2
  Subtract_cb1bc/1 -> Divide_d1542/2
  Constant_x_l_b5fbc/1 -> Subtract_0262a/2
  Constant_x_qd_55fd7/1 -> Subtract_02e5a/1
  Constant_-1_3da43/1 -> Product_40773/1
  Subtract_cc85e/1 -> Divide_51fce/2
  Constant_x_l_f3b31/1 -> Product_40773/2
  Product_f93d2/1 -> Divide_51fce/1
  Constant_-1_1a5f0/1 -> Product_3863b/1
  Product_3863b/1 -> Product_f93d2/1
  Constant_x_dd_9bd23/1 -> Subtract_277e5/1
  Constant_x_ddd_a9188/1 -> Subtract_277e5/2
  Add_5537a/1 -> Blockout_T_e_SG_D_3_4c18a/1
  State_psi_gq_SG_D_3_33d2c/1 -> Product_3102b/1
  Product_4afca/1 -> Divide_0d433/1
  Add_4be3a/1 -> Product_3102b/2
  State_psi_fd_SG_D_3_03760/1 -> Product_07c94/1
  Product_ae01e/1 -> Add_52871/1
  Constant_x_qd_c058a/1 -> Add_52871/2
  Constant_x_dd_2b2ae/1 -> Subtract_cc85e/1
  State_psi_kq_SG_D_3_78f61/1 -> Product_16dfe/1
  Constant_x_dd_ff414/1 -> Subtract_cb1bc/1
  Subtract_02e5a/1 -> Product_16dfe/2
  Product_7b82c/1 -> Divide_2e403/1
  Product_40773/1 -> Add_9b82a/1
  Add_52871/1 -> Divide_f1a46/2
  Constant_x_qd_eba46/1 -> Add_9b82a/2
  Subtract_277e5/1 -> Product_f93d2/2
  Constant_x_l_2b5e6/1 -> Subtract_cc85e/2
  Constant_x_ddd_f68ef/1 -> Subtract_0262a/1
  Product_3102b/1 -> Divide_f1a46/1
  Product_16dfe/1 -> Divide_4b437/1
  Add_9b82a/1 -> Divide_4b437/2
  Constant_x_ddd_00f81/1 -> Divide_0d433/2
  Subtract_0262a/1 -> Product_07c94/2
  Divide_f1a46/1 -> Subtract_ad55d/1
  Constant_x_l_58231/1 -> Subtract_cb1bc/2
  Divide_4b437/1 -> Subtract_ad55d/2
  Divide_51fce/1 -> Add_ba54b/1
  Product_07c94/1 -> Divide_d1542/1
  Constant_-1_81735/1 -> Product_8cdad/1
  State_psi_d_SG_D_3_21043/1 -> Product_8cdad/2
  Subtract_ad55d/1 -> Add_d82aa/1
  Divide_d1542/1 -> Subtract_1ae10/2
  Product_8cdad/1 -> Product_7b82c/1
  Constant_x_qdd_73938/1 -> Divide_2e403/2
  Divide_2e403/1 -> Add_5537a/1
  Divide_0d433/1 -> Add_5537a/2

== system case7/SG_D_3/d_E_fd_SG_D_3_block ==
  note: d_E_fd_SG_D_3 in case7
      | $\frac{V_{f,\mathrm{SG},D,3}-E_{\mathrm{fd},\mathrm{SG},D,3}\,K_{E}}{T_{E}}$
      | Automatically generated on 2025-10-31 19:26:16 .
  State_E_fd_SG_D_3_e3ff2 : Inport
  State_V_f_SG_D_3_f0dc9 : Inport  Port=2
  Add_95f26 : Sum
  Constant_-1_c5216 : Constant  Value=-1
  Constant_K_E_4c54a : Constant  Value=K_E
  Constant_T_E_0aeb7 : Constant  Value=T_E
  Divide_47da3 : Product  Inputs=*/
  Product_4f1a1 : Product
  Product_9169b : Product
  Blockout_d_E_fd_SG_D_3_4637c : Outport
  wires:
  State_V_f_SG_D_3_f0dc9/1 -> Add_95f26/2
  Constant_-1_c5216/1 -> Product_9169b/1
  State_E_fd_SG_D_3_e3ff2/1 -> Product_9169b/2
  Constant_T_E_0aeb7/1 -> Divide_47da3/2
  Product_9169b/1 -> Product_4f1a1/1
  Product_4f1a1/1 -> Add_95f26/1
  Constant_K_E_4c54a/1 -> Product_4f1a1/2
  Divide_47da3/1 -> Blockout_d_E_fd_SG_D_3_4637c/1
  Add_95f26/1 -> Divide_47da3/1

== system case7/SG_D_3/d_Px_1_SG_D_3_block ==
  note: d_Px_1_SG_D_3 in case7
      | $\frac{w_{\mathrm{SG},D,3}-2\,\pi \,f_{0}}{T_{w}}-\frac{\mathrm{Px}_{1,\mathrm{SG},D,3}}{T_{w}}$
      | Automatically generated on 2025-10-31 19:26:18 .
  State_Px_1_SG_D_3_f55d0 : Inport
  State_w_SG_D_3_68398 : Inport  Port=2
  Add_cc710 : Sum
  Add_e78cc : Sum
  Constant_-1_850ec : Constant  Value=-1
  Constant_-2.0_7280e : Constant  Value=-2.0
  Constant_T_w_2334b : Constant  Value=T_w
  Constant_T_w_8c660 : Constant  Value=T_w
  Constant_f0_8097a : Constant  Value=f0
  Constant_pi_cadd3 : Constant  Value=pi
  Divide_49863 : Product  Inputs=*/
  Divide_a18ee : Product  Inputs=*/
  Product_57517 : Product
  Product_806a6 : Product
  Product_e016d : Product
  Blockout_d_Px_1_SG_D_3_f80fa : Outport
  wires:
  Constant_f0_8097a/1 -> Product_57517/2
  Constant_-1_850ec/1 -> Product_e016d/1
  Constant_-2.0_7280e/1 -> Product_806a6/1
  Constant_pi_cadd3/1 -> Product_806a6/2
  Product_806a6/1 -> Product_57517/1
  State_w_SG_D_3_68398/1 -> Add_cc710/2
  Divide_a18ee/1 -> Add_e78cc/1
  State_Px_1_SG_D_3_f55d0/1 -> Product_e016d/2
  Product_57517/1 -> Add_cc710/1
  Product_e016d/1 -> Divide_a18ee/1
  Constant_T_w_2334b/1 -> Divide_a18ee/2
  Add_cc710/1 -> Divide_49863/1
  Constant_T_w_8c660/1 -> Divide_49863/2
  Divide_49863/1 -> Add_e78cc/2
  Add_e78cc/1 -> Blockout_d_Px_1_SG_D_3_f80fa/1

== system case7/SG_D_3/d_Px_2_SG_D_3_block ==
  note: d_Px_2_SG_D_3 in case7
      | $\frac{\mathrm{Px}_{1,\mathrm{SG},D,3}-T_{2}\,\left(\frac{\mathrm{Px}_{1,\mathrm{SG},D,3}}{T_{w}}-\frac{w_{\mathrm{SG},D,3}-2\,\pi \,f_{0}}{T_{w}}\right)}{T_{1}}-\frac{\mathrm{Px}_{2,\mathrm{SG},D,3}}{T_{1}}$
      | Automatically generated on 2025-10-31 19:26:20 .
  State_Px_2_SG_D_3_db3bd : Inport
  State_Px_1_SG_D_3_910c8 : Inport  Port=2
  State_Px_1_SG_D_3_d78a2 : Inport  Port=3
  State_w_SG_D_3_fe34a : Inport  Port=4
  Add_5b373 : Sum
  Add_6d838 : Sum
  Add_e0d6c : Sum
  Add_e9346 : Sum
  Constant_-1_989ae : Constant  Value=-1
  Constant_-1_aa5fc : Constant  Value=-1
  Constant_-2.0_cb4b5 : Constant  Value=-2.0
  Constant_T_1_08c33 : Constant  Value=T_1
  Constant_T_1_a267c : Constant  Value=T_1
  Constant_T_2_0fb1f : Constant  Value=T_2
  Constant_T_w_a57ad : Constant  Value=T_w
  Constant_T_w_c2254 : Constant  Value=T_w
  Constant_f0_f3284 : Constant  Value=f0
  Constant_pi_38d0f : Constant  Value=pi
  Divide_33ee8 : Product  Inputs=*/
  Divide_43a20 : Product  Inputs=*/
  Divide_95663 : Product  Inputs=*/
  Divide_ee43b : Product  Inputs=*/
  Product_17bd3 : Product
  Product_1e82b : Product
  Product_26dd2 : Product
  Product_97bfa : Product
  Product_da245 : Product
  Blockout_d_Px_2_SG_D_3_8d5d5 : Outport
  wires:
  State_Px_1_SG_D_3_d78a2/1 -> Product_17bd3/2
  Constant_-2.0_cb4b5/1 -> Product_1e82b/1
  Constant_f0_f3284/1 -> Product_26dd2/2
  Constant_pi_38d0f/1 -> Product_1e82b/2
  Product_1e82b/1 -> Product_26dd2/1
  State_w_SG_D_3_fe34a/1 -> Add_e0d6c/2
  Constant_-1_989ae/1 -> Product_17bd3/1
  Product_26dd2/1 -> Add_e0d6c/1
  Product_17bd3/1 -> Divide_33ee8/1
  Constant_T_w_c2254/1 -> Divide_33ee8/2
  Add_e0d6c/1 -> Divide_ee43b/1
  Constant_T_w_a57ad/1 -> Divide_ee43b/2
  Divide_33ee8/1 -> Add_5b373/1
  Divide_ee43b/1 -> Add_5b373/2
  Constant_T_2_0fb1f/1 -> Product_da245/1
  Add_5b373/1 -> Product_da245/2
  Constant_-1_aa5fc/1 -> Product_97bfa/1
  Product_da245/1 -> Add_e9346/2
  State_Px_2_SG_D_3_db3bd/1 -> Product_97bfa/2
  State_Px_1_SG_D_3_910c8/1 -> Add_e9346/1
  Product_97bfa/1 -> Divide_95663/1
  Add_6d838/1 -> Blockout_d_Px_2_SG_D_3_8d5d5/1
  Constant_T_1_a267c/1 -> Divide_95663/2
  Add_e9346/1 -> Divide_43a20/1
  Constant_T_1_08c33/1 -> Divide_43a20/2
  Divide_95663/1 -> Add_6d838/1
  Divide_43a20/1 -> Add_6d838/2

== system case7/SG_D_3/d_Px_3_SG_D_3_block ==
  note: d_Px_3_SG_D_3 in case7
      | $\frac{\mathrm{Px}_{2,\mathrm{SG},D,3}+T_{4}\,\left(\frac{\mathrm{Px}_{1,\mathrm{SG},D,3}-T_{2}\,\left(\frac{\mathrm{Px}_{1,\mathrm{SG},D,3}}{T_{w}}-\frac{w_{\mathrm{SG},D,3}-2\,\pi \,f_{0}}{T_{w}}\right)}{T_{1}}-\frac{\mathrm{Px}_{2,\mathrm{SG},D,3}}{T_{1}}\right)}{T_{3}}-\frac{\mathrm{Px}_{3,\mathrm{SG},D,3}}{T_{3}}$
      | Automatically generated on 2025-10-31 19:26:23 .
  State_Px_3_SG_D_3_8e084 : Inport
  State_Px_2_SG_D_3_e7342 : Inport  Port=2
  State_Px_2_SG_D_3_4c474 : Inport  Port=3
  State_Px_1_SG_D_3_9cfb8 : Inport  Port=4
  State_Px_1_SG_D_3_6302b : Inport  Port=5
  State_w_SG_D_3_03f21 : Inport  Port=6
  Add_1ee13 : Sum
  Add_8b109 : Sum
  Add_8f57e : Sum
  Add_9ced1 : Sum
  Add_c30c3 : Sum
  Add_edbee : Sum
  Constant_-1_4b5a3 : Constant  Value=-1
  Constant_-1_75ca0 : Constant  Value=-1
  Constant_-1_8dec9 : Constant  Value=-1
  Constant_-2.0_25459 : Constant  Value=-2.0
  Constant_T_1_03730 : Constant  Value=T_1
  Constant_T_1_0914d : Constant  Value=T_1
  Constant_T_2_47f2a : Constant  Value=T_2
  Constant_T_3_5a699 : Constant  Value=T_3
  Constant_T_3_e4c83 : Constant  Value=T_3
  Constant_T_4_183ff : Constant  Value=T_4
  Constant_T_w_156ad : Constant  Value=T_w
  Constant_T_w_29fd3 : Constant  Value=T_w
  Constant_f0_4667f : Constant  Value=f0
  Constant_pi_affe4 : Constant  Value=pi
  Divide_03936 : Product  Inputs=*/
  Divide_6c80d : Product  Inputs=*/
  Divide_77c6f : Product  Inputs=*/
  Divide_bdd48 : Product  Inputs=*/
  Divide_beb66 : Product  Inputs=*/
  Divide_cdf68 : Product  Inputs=*/
  Product_3074a : Product
  Product_7d19d : Product
  Product_82df0 : Product
  Product_d5dc0 : Product
  Product_d93fe : Product
  Product_f18e1 : Product
  Product_fe44d : Product
  Blockout_d_Px_3_SG_D_3_7ae60 : Outport
  wires:
  State_Px_1_SG_D_3_6302b/1 -> Product_d93fe/2
  Constant_f0_4667f/1 -> Product_f18e1/2
  Constant_-2.0_25459/1 -> Product_82df0/1
  Add_9ced1/1 -> Divide_77c6f/1
  Constant_pi_affe4/1 -> Product_82df0/2
  Product_82df0/1 -> Product_f18e1/1
  State_w_SG_D_3_03f21/1 -> Add_8b109/2
  Constant_T_w_29fd3/1 -> Divide_03936/2
  Constant_-1_75ca0/1 -> Product_d93fe/1
  Product_f18e1/1 -> Add_8b109/1
  Product_d93fe/1 -> Divide_03936/1
  Add_8b109/1 -> Divide_cdf68/1
  Product_d5dc0/1 -> Divide_6c80d/1
  Constant_T_w_156ad/1 -> Divide_cdf68/2
  Divide_03936/1 -> Add_8f57e/1
  Divide_cdf68/1 -> Add_8f57e/2
  Constant_T_2_47f2a/1 -> Product_fe44d/1
  Add_8f57e/1 -> Product_fe44d/2
  Constant_-1_8dec9/1 -> Product_d5dc0/1
  State_Px_2_SG_D_3_4c474/1 -> Product_d5dc0/2
  State_Px_1_SG_D_3_9cfb8/1 -> Add_9ced1/1
  Constant_T_3_5a699/1 -> Divide_bdd48/2
  Product_fe44d/1 -> Add_9ced1/2
  Constant_T_1_0914d/1 -> Divide_6c80d/2
  Add_c30c3/1 -> Product_7d19d/2
  Constant_T_1_03730/1 -> Divide_77c6f/2
  Divide_beb66/1 -> Add_1ee13/2
  Divide_6c80d/1 -> Add_c30c3/1
  Divide_77c6f/1 -> Add_c30c3/2
  Constant_T_4_183ff/1 -> Product_7d19d/1
  Constant_-1_4b5a3/1 -> Product_3074a/1
  State_Px_3_SG_D_3_8e084/1 -> Product_3074a/2
  State_Px_2_SG_D_3_e7342/1 -> Add_edbee/1
  Product_7d19d/1 -> Add_edbee/2
  Product_3074a/1 -> Divide_bdd48/1
  Add_edbee/1 -> Divide_beb66/1
  Constant_T_3_e4c83/1 -> Divide_beb66/2
  Divide_bdd48/1 -> Add_1ee13/1
  Add_1ee13/1 -> Blockout_d_Px_3_SG_D_3_7ae60/1
